simulink model "clasificador_armonicos"  (R2017b)
settings: Solver=VariableStepAuto  StartTime=0.0  StopTime=10  RelTol=1e-3
settings Model: Creator=choqi  LastModifiedBy=choqi

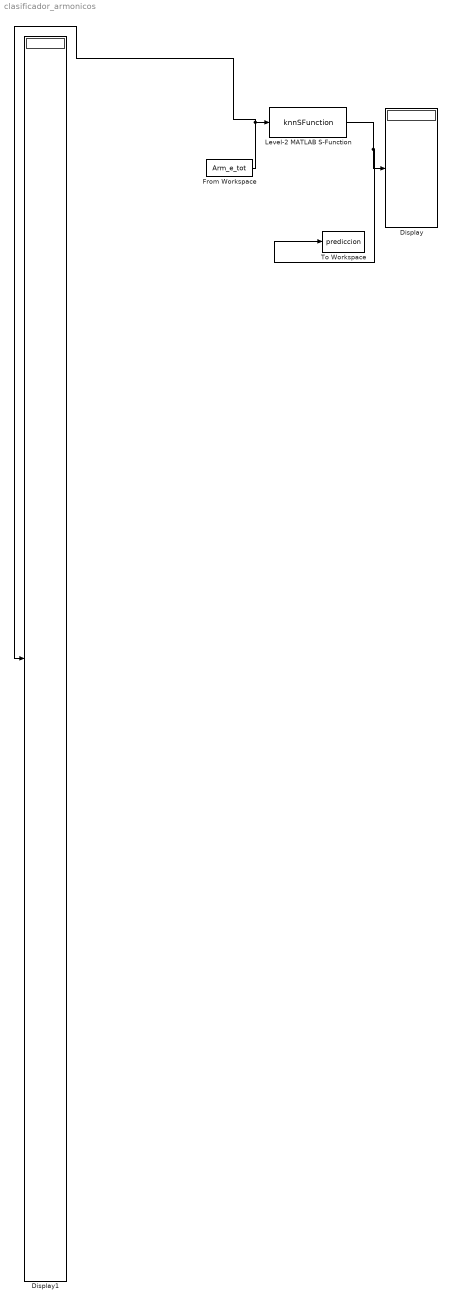
== system clasificador_armonicos ==
  Display : Display
  Display1 : Display
  From Workspace : FromWorkspace  VariableName=Arm_e_tot  SampleTime=0
  Level-2 MATLAB S-Function : M-S-Function  FunctionName=knnSFunction
  To Workspace : ToWorkspace  VariableName=prediccion  SampleTime=-1
      settings: Save2DSignal=2-D array (concatenate along first dimension)
  wires:
  Level-2 MATLAB S-Function/1 -> To Workspace/1, Display/1
  From Workspace/1 -> Display1/1, Level-2 MATLAB S-Function/1
